simulink model "sdrzQPSKRxFPGA"  (R2016a)
settings: Solver=FixedStepDiscrete  SolverMode=SingleTasking  StartTime=0.0  StopTime=Inf  RelTol=1e-3
PreLoadFcn:
  | sdrzQPSKrxFPGA = sdrzQPSKRxFPGA_init;
InitFcn:
  | sdrzQPSKrxFPGA = sdrzQPSKRxFPGA_init;
libraries: hdlsllib x4, dspsigops x2, simulink x2, sdrzblksprivate x1, commsequence2 x1, dspmathops x1, commdigbbndpm3 x1, dspmlti4 x1, sdrzlib x1
CloseFcn:
  | clear sdrzQPSKrxFPGA;
Description:
  | This model is used to generate a targeted .bit for an SDR platform
settings Model: FPTRunName=Active  ModifiedByFormat=The MathWorks Inc.  SimulationMode=accelerator  Creator=The MathWorks, Inc.  LastModifiedBy=The MathWorks Inc.
settings DataIOCC: LimitDataPoints=on  SaveFormat=Structure  SaveOutput=off  SignalLogging=off  DSMLogging=off  SaveTime=off
settings OptimizationCC: BlockReduction=off  ConditionallyExecuteInputs=off  DefaultParameterBehavior=Inlined  ExpressionDepthLimit=2147483647  LocalBlockOutputs=off  SimCompilerOptimization=on
settings DebuggingCC: AlgebraicLoopMsg=error  UnderspecifiedInitializationDetection=Classic  MergeDetectMultiDrivingBlocksExec=none  SolverPrmCheckMsg=warning  MultiTaskDSMMsg=warning  MultiTaskCondExecSysMsg=none  SingleTaskRateTransMsg=error  ParameterPrecisionLossMsg=none  FcnCallInpInsideContextMsg=UseLocalSettings  AllowSymbolicDim=off  StateNameClashWarn=warning
settings HardwareCC: ProdBitPerPointer=32  ProdLargestAtomicFloat=None  ProdIntDivRoundTo=Undefined  ProdEndianess=Unspecified  ProdWordSize=32  ProdHWDeviceType=ASIC/FPGA->ASIC/FPGA  TargetBitPerPointer=64  TargetLongLongMode=on  TargetIntDivRoundTo=Zero  TargetEndianess=LittleEndian  TargetWordSize=64  TargetHWDeviceType=MATLAB Host  ProdEqTarget=off
settings ModelReferenceCC: PropagateSignalLabelsOutOfModel=off
settings RTWCC: CustomSourceCode=|
  | #include <stdio.h>
  | #include <stdlib.h>
settings GRTTargetCC: CombineOutputUpdateFcns=off  GRTInterface=on
settings ConfigComp: CovModelRefEnable=Off  CovSFcnEnable=off

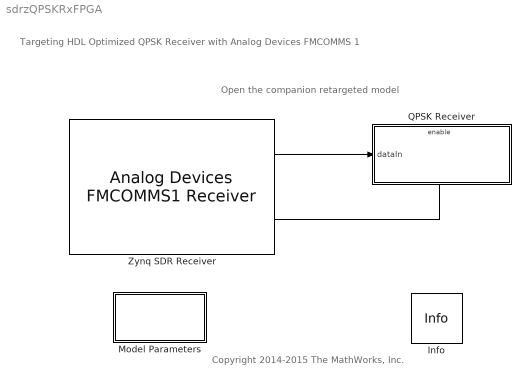
== system sdrzQPSKRxFPGA ==
  note: Copyright 2014-2015 The MathWorks, Inc.
  note: Targeting HDL Optimized QPSK Receiver with Analog Devices FMCOMMS 1
  note: Open the companion retargeted model
  Info : sdrzblksprivate/Info  SystemSampleTime=-1
  Model Parameters : Subsystem  mask(Model Parameters){SettingCtrl=Automatic gain control settings, AutoGainCtrlLoopGain=0.1, AutoGainCtrlMaxGain=400, FineFreqNormalizedLoopBW=0.06, FineFreqDampingFactor=2.5, TimeRecNormalizedLoopBW=0.01, TimeRecDampingFactor=1, DataDecThreshold=16}
      mask prompts: SettingCtrl "Setting type:"; AutoGainCtrlLoopGain "Loop gain:"; AutoGainCtrlMaxGain "Gain upper limit:"; FineFreqNormalizedLoopBW "Normalized loop bandwidth:"; FineFreqDampingFactor "Damping factor:"; TimeRecNormalizedLoopBW "Normalized loop bandwidth:"; TimeRecDampingFactor "Damping factor:"; DataDecThreshold "Threshold for the modulus of the Matched Filter ouput:"
      mask help: Set parameters for the QPSK receiver model
      mask init:
      | myException = sdrzQPSKRxFPGA_mask(gcb, 'init');
      | if ~isempty(myException)
      |    errordlg(myException.msg);
      | end
      mask TypeOptions SettingCtrl: Automatic gain control settings | Fine frequency compensation settings | Timing recovery settings | Data decoding settings
      mask Callback SettingCtrl: sdrzQPSKRxFPGA_mask(gcbh, 'cbShowHideSettingOptions');
      mask Display: disp('Model\nParameters');
  QPSK Receiver : Subsystem
      mask Display: disp('QPSK Receiver')
  Zynq SDR Receiver : sdrzlib/Analog Devices FMCOMMS1 Receiver  SourceLibraryInfo="This block requires Communications System Toolbox Support Package for Xilinx FPGA-Based Radio. <a href=\"http://www.mathworks.com/hardware-support-packages\">More information</a>"  sobjType=comm.SDRZynqFMCOMMS1Receiver  IPAddress=192.168.3.2  dataUDPPort=-1  ctrlUDPPort=-1  subDeviceList=comm.SDRZynqFMCOMMS1Receiver  sdrBlockType=SDRBlockTypeSLT.SDRRxBlock  requester=UNUSED_BY_SFCN  sdrExecutionMode=HW  LostSamplesOutputPort=off  OutputDataType=double  FrameLength=sdrzQPSKrxFPGA.Upsampling*sdrzQPSKrxFPGA.FrameSize*sdrzQPSKrxFPGA.RxBufferedFrames  EnableBurstMode=on  NumFramesInBurst=500  BypassUserLogic=on  DecimatorSelect=DDC decimator  SourceSelect=RF data  SineAmplitude=16000  SineFrequency=30000  EnableInternalClock=off  BypassIQBalance=on  CenterFrequencySource=Dialog  CenterFrequency=sdrzQPSKrxFPGA.RadioCenterFrequency  IntermediateFrequencySource=Dialog  IntermediateFrequency=sdrzQPSKrxFPGA.RadioIntermediateFrequency  IFBandwidthSource=Dialog  IFBandwidth=40e6  ADCRateSource=Dialog  ADCRate=sdrzQPSKrxFPGA.RadioADCRate  GainSource=Dialog  Gain=sdrzQPSKrxFPGA.RadioGain  DecimationFactorSource=Dialog  DecimationFactor=sdrzQPSKrxFPGA.RadioDecimationFactor  RFFrequencyIsTunable=logical(0)  SampleTime=sdrzQPSKrxFPGA.Ts  BypassDCBlockingFilter=off  IQBalanceCoefficients=64  SkipAllHardwareResetAndInitialization=off  EnableIQCalibrationTable=on  CacheIQCalibrationTable=off
  wires:
  Zynq SDR Receiver/1 -> QPSK Receiver/1(dataIn)
  Zynq SDR Receiver/2 -> QPSK Receiver/Enable

== system sdrzQPSKRxFPGA/Model Parameters ==

== system sdrzQPSKRxFPGA/QPSK Receiver ==
  dataIn : Inport  OutDataTypeStr=double
  Enable : EnablePort
  " " : MATLAB Function  TreatAsAtomicUnit=on
  Buffer1 : Buffer  N=4000  TreatMby1Signals=One channel  OutputFrames=off
  Data Type Conversion1 : DataTypeConversion  OutDataTypeStr=fixdt(1,16,15)
  Descramble and Print : Subsystem  TreatAsAtomicUnit=on
  HDLRx : Subsystem
  Unbuffer : Unbuffer  SampleBasedProcessing=Same as frame based
  Unpack FPGA Outputs : Subsystem
  wires:
  dataIn/1 -> Data Type Conversion1/1
  Unpack FPGA Outputs/2(bit2) -> " "/2(bit2)
  Unpack FPGA Outputs/1(bit1) -> " "/1(bit1)
  Unpack FPGA Outputs/3(dValid) -> " "/3(datavld)
  Buffer1/1 -> Unpack FPGA Outputs/1(In1)
  HDLRx/1(out) -> Buffer1/1
  Data Type Conversion1/1 -> Unbuffer/1
  Unbuffer/1 -> HDLRx/1(dataIn)
  " "/1(RxGo) -> Descramble and Print/Enable
  " "/2(framed_data) -> Descramble and Print/1(In1)

== system sdrzQPSKRxFPGA/QPSK Receiver/Descramble and Print ==
  In1 : Inport
  Enable : EnablePort
  BitsToDecimal1 : MATLAB Function  TreatAsAtomicUnit=on
  Buffer : Buffer  N=200  TreatMby1Signals=One channel  OutputFrames=off
  Descrambling : Subsystem
      mask Display: disp('Descrambling')
  wires:
  Descrambling/1(Out) -> BitsToDecimal1/1(u)
  In1/1 -> Buffer/1
  Buffer/1 -> Descrambling/1(In)

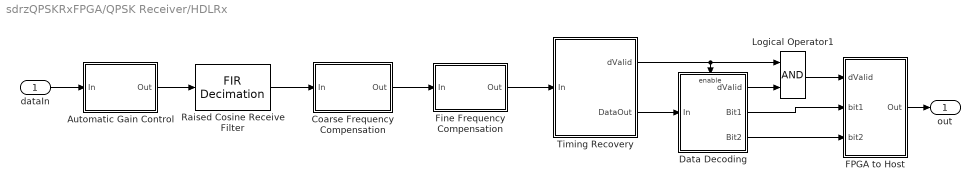
== system sdrzQPSKRxFPGA/QPSK Receiver/HDLRx ==
  dataIn : Inport
  Automatic Gain Control : Subsystem  mask{AGCLoopGain=0.1, AGCUpperLimit=400, AGCRef=1/sqrt(sdrzQPSKrxFPGA.Upsampling)}
      mask prompts: AGCLoopGain "Loop Gain"; AGCUpperLimit "Maximum Gain"; AGCRef "Desired Amplitude"
  Coarse Frequency Compensation : Subsystem
  Data Decoding : Subsystem  TreatAsAtomicUnit=on  mask{Threshold=16}
      mask help:
      | Package synchronization is achieved by correlating (matched filtering) the Barker codes with the streams given by the Timing Recovery subsystem.
      | We deem successful package synchronization if the modulus of the matched filter output exceeds the threshold value defined below.
  FPGA to Host : Subsystem
  Fine Frequency Compensation : Subsystem
  Logical Operator1 : Logic  AllPortsSameDT=off  OutDataTypeStr=boolean
  Raised Cosine Receive Filter : dspmlti4/FIR Decimation  FilterSource=Dialog parameters  h=sdrzQPSKrxFPGA.ReceiverFilterCoefficients  D=sdrzQPSKrxFPGA.Upsampling/sdrzQPSKrxFPGA.Downsampling  filtStruct=Direct form  FilterObject=Hm_firdecim  framing=Allow multirate processing  inputOffset=0  outputBufInitCond=0  roundingMode=Floor  overflowMode=off  firstCoeffDataTypeStr=Inherit: Same word length as input  firstCoeffMin=[]  firstCoeffMax=[]  firstCoeffLastDataTypeStr=Inherit: Same word length as input  outputMode=Binary point scaling  outputWordLength=16  outputFracLength=14  outputDataTypeStr=fixdt(1,16,14)  outputMin=[]  outputMax=[]  outputLastDataTypeStr=fixdt(1,16,14)
  Timing Recovery : Subsystem
  out : Outport
  wires:
  Timing Recovery/2(DataOut) -> Data Decoding/1(In)
  dataIn/1 -> Automatic Gain Control/1(In)
  Fine Frequency Compensation/1(Out) -> Timing Recovery/1(In)
  Coarse Frequency Compensation/1(Out) -> Fine Frequency Compensation/1(In)
  Timing Recovery/1(dValid) -> Logical Operator1/1, Data Decoding/Enable
  Data Decoding/1(dValid) -> Logical Operator1/2
  Raised Cosine Receive Filter/1 -> Coarse Frequency Compensation/1(In)
  Automatic Gain Control/1(Out) -> Raised Cosine Receive Filter/1
  Logical Operator1/1 -> FPGA to Host/1(dValid)
  Data Decoding/3(Bit2) -> FPGA to Host/3(bit2)
  Data Decoding/2(Bit1) -> FPGA to Host/2(bit1)
  FPGA to Host/1(Out) -> out/1

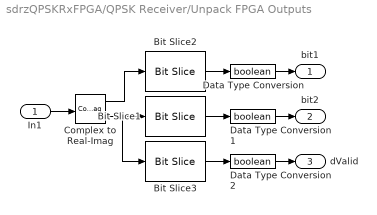
== system sdrzQPSKRxFPGA/QPSK Receiver/Unpack FPGA Outputs ==
  In1 : Inport
  Bit Slice1 : hdlsllib/HDL Operations/Bit Slice  lidx=0  ridx=0
  Bit Slice2 : hdlsllib/HDL Operations/Bit Slice  lidx=0  ridx=0
  Bit Slice3 : hdlsllib/HDL Operations/Bit Slice  lidx=15  ridx=15
  Complex to Real-Imag : ComplexToRealImag
  Data Type Conversion : DataTypeConversion  OutDataTypeStr=boolean
  Data Type Conversion1 : DataTypeConversion  OutDataTypeStr=boolean
  Data Type Conversion2 : DataTypeConversion  OutDataTypeStr=boolean
  bit1 : Outport
  bit2 : Outport  Port=2
  dValid : Outport  Port=3
  wires:
  In1/1 -> Complex to Real-Imag/1
  Complex to Real-Imag/1 -> Bit Slice2/1
  Complex to Real-Imag/2 -> Bit Slice3/1, Bit Slice1/1
  Bit Slice2/1 -> Data Type Conversion/1
  Bit Slice1/1 -> Data Type Conversion1/1
  Bit Slice3/1 -> Data Type Conversion2/1
  Data Type Conversion/1 -> bit1/1
  Data Type Conversion1/1 -> bit2/1
  Data Type Conversion2/1 -> dValid/1

== system sdrzQPSKRxFPGA/QPSK Receiver/Descramble and Print/Descrambling ==
  In : Inport
  Descrambler : commsequence2/Descrambler  M=2  poly=[1 1 1 0 1]  iniStaSource=Dialog Parameter  ini_sta=[0 0 0 0]  resetViaPort=off
  Selector : Selector  IndexOptions=Index vector (dialog)  Indices=[sdrzQPSKrxFPGA.BarkerLength*log2(sdrzQPSKrxFPGA.M)+1:sdrzQPSKrxFPGA.FrameSize*log2(sdrzQPSKrxFPGA.M)]  OutputSizes=1
  Selector1 : Selector  IndexOptions=Index vector (dialog)  Indices=[1:sdrzQPSKrxFPGA.MsgLength]  OutputSizes=1
  Out : Outport
  wires:
  Descrambler/1 -> Selector1/1
  Selector1/1 -> Out/1
  In/1 -> Selector/1
  Selector/1 -> Descrambler/1

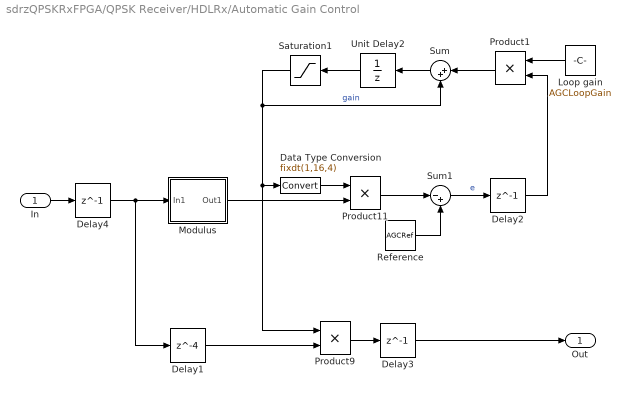
== system sdrzQPSKRxFPGA/QPSK Receiver/HDLRx/Automatic Gain Control ==
  In : Inport
  Data Type Conversion : DataTypeConversion  OutDataTypeStr=fixdt(1,16,4)  SaturateOnIntegerOverflow=on
  Delay1 : Delay  DelayLength=4  InitialCondition=0
  Delay2 : Delay  DelayLength=1  InitialCondition=0
  Delay3 : Delay  DelayLength=1  InitialCondition=0
  Delay4 : Delay  DelayLength=1  InitialCondition=0
  Loop gain : Constant  Value=AGCLoopGain  OutDataTypeStr=fixdt(1,16,10)  SampleTime=sdrzQPSKrxFPGA.Ts
  Modulus : Subsystem
  Product1 : Product  OutDataTypeStr=fixdt(1,16,10)  RndMeth=Zero
  Product11 : Product  OutDataTypeStr=fixdt(1,16,10)  RndMeth=Zero
  Product9 : Product  OutDataTypeStr=fixdt(1,16,14)  SaturateOnIntegerOverflow=on  RndMeth=Zero
  Reference : Constant  Value=AGCRef  OutDataTypeStr=fixdt(1,16,10)  SampleTime=sdrzQPSKrxFPGA.Ts
  Saturation1 : Saturate  UpperLimit=AGCUpperLimit  LowerLimit=1e-5
  Sum : Sum  Inputs=|++  OutDataTypeStr=fixdt(1,23,10)  SaturateOnIntegerOverflow=on
  Sum1 : Sum  Inputs=|-+  OutDataTypeStr=Inherit: Same as first input
  Unit Delay2 : UnitDelay  SampleTime=-1
  Out : Outport  PortDimensions=1
  wires:
  In/1 -> Delay4/1
  Product11/1 -> Sum1/1
  Data Type Conversion/1 -> Product11/1
  Reference/1 -> Sum1/2
  Sum/1 -> Unit Delay2/1
  Sum1/1 -> Delay2/1  "e"
  Product9/1 -> Delay3/1
  Delay1/1 -> Product9/2
  Delay3/1 -> Out/1
  Delay2/1 -> Product1/2
  Unit Delay2/1 -> Saturation1/1
  Delay4/1 -> Delay1/1, Modulus/1(In1)
  Modulus/1(Out1) -> Product11/2
  Product1/1 -> Sum/1
  Loop gain/1 -> Product1/1
  Saturation1/1 -> Sum/2, Data Type Conversion/1, Product9/1  "gain"

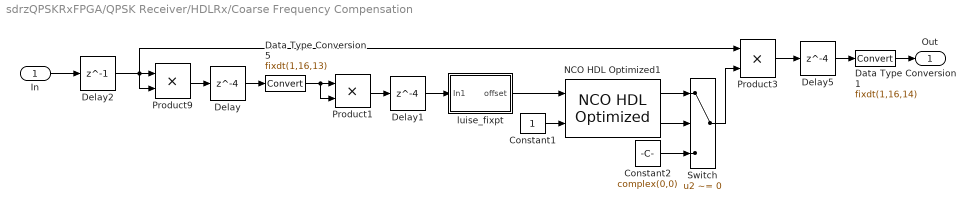
== system sdrzQPSKRxFPGA/QPSK Receiver/HDLRx/Coarse Frequency Compensation ==
  In : Inport  PortDimensions=1
  Constant1 : Constant  OutDataTypeStr=boolean  SampleTime=sdrzQPSKrxFPGA.Ts*sdrzQPSKrxFPGA.Upsampling/sdrzQPSKrxFPGA.Downsampling
  Constant2 : Constant  Value=complex(0,0)  OutDataTypeStr=fixdt(1,10,8)  SampleTime=sdrzQPSKrxFPGA.Ts*sdrzQPSKrxFPGA.Upsampling/sdrzQPSKrxFPGA.Downsampling
  Data Type Conversion1 : DataTypeConversion  OutDataTypeStr=fixdt(1,16,14)
  Data Type Conversion5 : DataTypeConversion  OutDataTypeStr=fixdt(1,16,13)  SaturateOnIntegerOverflow=on
  Delay : Delay  DelayLength=4  InitialCondition=0
  Delay1 : Delay  DelayLength=4  InitialCondition=0
  Delay2 : Delay  DelayLength=1  InitialCondition=0
  Delay5 : Delay  DelayLength=4  InitialCondition=0
  NCO HDL Optimized1 : dspsigops/NCO HDL Optimized  PhaseIncrementSource=Input port  PhaseIncrement=100  PhaseOffsetSource=Property  PhaseOffset=0  DitherSource=None  NumDitherBits=1  PhaseQuantization=on  NumQuantizerAccumulatorBits=16  LUTCompress=on  ResetAction=off  ValidInputPort=on  Waveform=Complex exponential  PhasePort=off  AccumulatorWL=17  OutputDataType=Binary point scaling  OutputWL=10  OutputFL=8  SimulateUsing=Code generation
  Product1 : Product  SaturateOnIntegerOverflow=on  RndMeth=Zero
  Product3 : Product  SaturateOnIntegerOverflow=on  RndMeth=Zero
  Product9 : Product  SaturateOnIntegerOverflow=on  RndMeth=Zero
  Switch : Switch  Criteria=u2 ~= 0
  luise_fixpt : Subsystem
  Out : Outport
  wires:
  Data Type Conversion1/1 -> Out/1
  Delay1/1 -> luise_fixpt/1(In1)
  Product9/1 -> Delay/1
  Delay/1 -> Data Type Conversion5/1
  Data Type Conversion5/1 -> Product1/1, Product1/2
  Product1/1 -> Delay1/1
  In/1 -> Delay2/1
  Product3/1 -> Delay5/1
  Delay5/1 -> Data Type Conversion1/1
  Constant1/1 -> NCO HDL Optimized1/2
  NCO HDL Optimized1/2 -> Switch/2
  NCO HDL Optimized1/1 -> Switch/1
  Constant2/1 -> Switch/3
  Switch/1 -> Product3/2
  Delay2/1 -> Product3/1, Product9/2, Product9/1
  luise_fixpt/1(offset) -> NCO HDL Optimized1/1

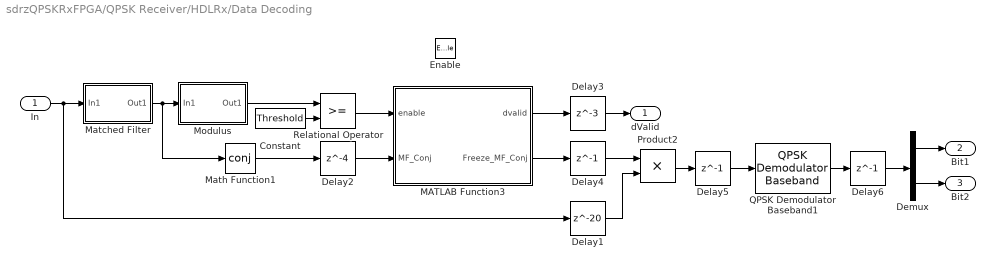
== system sdrzQPSKRxFPGA/QPSK Receiver/HDLRx/Data Decoding ==
  In : Inport
  Enable : EnablePort
  Constant : Constant  Value=Threshold  OutDataTypeStr=Inherit: Inherit via back propagation  SampleTime=sdrzQPSKrxFPGA.Ts*sdrzQPSKrxFPGA.Upsampling/sdrzQPSKrxFPGA.Downsampling
  Delay1 : Delay  DelayLength=20  InitialCondition=0
  Delay2 : Delay  DelayLength=4  InitialCondition=0
  Delay3 : Delay  DelayLength=3  InitialCondition=0
  Delay4 : Delay  DelayLength=1  InitialCondition=0
  Delay5 : Delay  DelayLength=1  InitialCondition=0
  Delay6 : Delay  DelayLength=1  InitialCondition=0
  Demux : Demux  Outputs=2
  MATLAB Function3 : MATLAB Function  TreatAsAtomicUnit=on
  Matched Filter : Subsystem
  Math Function1 : Math  Operator=conj  OutputSignalType=complex  SaturateOnIntegerOverflow=on
  Modulus : Subsystem
  Product2 : Product  SaturateOnIntegerOverflow=on  RndMeth=Zero
  QPSK Demodulator Baseband1 : commdigbbndpm3/QPSK Demodulator Baseband  OutType=Bit  DecType=Hard decision  VarSource=Dialog  Variance=1  Dec=Gray  Ph=pi/4  outDtype1=boolean  outDtype2=Inherit via internal rule  derotateFactorWordLen=16  derotateFactorDataTypeStr=Inherit: Same word length as input  derotateFactorLastDataTypeStr=Inherit: Same word length as input
  Relational Operator : RelationalOperator  OutDataTypeStr=boolean  InputSameDT=on
  dValid : Outport  InitialOutput=0
  Bit1 : Outport  Port=2  InitialOutput=0
  Bit2 : Outport  Port=3  InitialOutput=0
  wires:
  Demux/2 -> Bit2/1
  Demux/1 -> Bit1/1
  Delay3/1 -> dValid/1
  Delay6/1 -> Demux/1
  Delay5/1 -> QPSK Demodulator Baseband1/1
  Delay1/1 -> Product2/2
  Delay4/1 -> Product2/1
  Delay2/1 -> MATLAB Function3/2(MF_Conj)
  Matched Filter/1(Out1) -> Math Function1/1, Modulus/1(In1)
  In/1 -> Delay1/1, Matched Filter/1(In1)
  Product2/1 -> Delay5/1
  Relational Operator/1 -> MATLAB Function3/1(enable)
  Math Function1/1 -> Delay2/1
  MATLAB Function3/2(Freeze_MF_Conj) -> Delay4/1
  MATLAB Function3/1(dvalid) -> Delay3/1
  QPSK Demodulator Baseband1/1 -> Delay6/1
  Modulus/1(Out1) -> Relational Operator/1
  Constant/1 -> Relational Operator/2

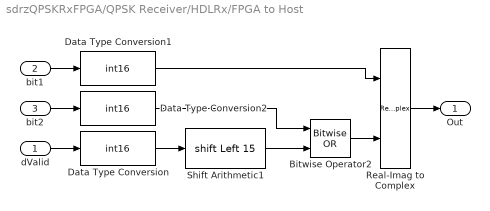
== system sdrzQPSKRxFPGA/QPSK Receiver/HDLRx/FPGA to Host ==
  dValid : Inport
  bit1 : Inport  Port=2
  bit2 : Inport  Port=3
  Bitwise Operator2 : simulink/Logic and Bit Operations/Bitwise Operator  logicop=OR  UseBitMask=off  NumInputPorts=2  BitMask=bin2dec('11011001')  BitMaskRealWorld=Stored Integer
  Data Type Conversion : DataTypeConversion  OutDataTypeStr=int16
  Data Type Conversion1 : DataTypeConversion  OutDataTypeStr=int16
  Data Type Conversion2 : DataTypeConversion  OutDataTypeStr=int16
  Real-Imag to Complex : RealImagToComplex
  Shift Arithmetic1 : ArithShift  BitShiftNumber=15  BitShiftDirection=Left
  Out : Outport
  wires:
  Data Type Conversion2/1 -> Bitwise Operator2/1
  Data Type Conversion1/1 -> Real-Imag to Complex/1
  Data Type Conversion/1 -> Shift Arithmetic1/1
  Real-Imag to Complex/1 -> Out/1
  bit2/1 -> Data Type Conversion2/1
  dValid/1 -> Data Type Conversion/1
  Bitwise Operator2/1 -> Real-Imag to Complex/2
  Shift Arithmetic1/1 -> Bitwise Operator2/2
  bit1/1 -> Data Type Conversion1/1

== system sdrzQPSKRxFPGA/QPSK Receiver/HDLRx/Fine Frequency Compensation ==
  In : Inport  PortDimensions=1
  Delay2 : Delay  DelayLength=1  InitialCondition=0
  Delay5 : Delay  DelayLength=9  InitialCondition=0
  Loop Filter : Subsystem  mask{BnTs=0.06, zeta=2.5, N=sdrzQPSKrxFPGA.Upsampling/sdrzQPSKrxFPGA.Downsampling, Kp=sdrzQPSKrxFPGA.FineFreqPEDGain, K0=sdrzQPSKrxFPGA.FineFreqCompensateGain}
      mask prompts: BnTs "Normalized Loop Bandwidth"; zeta "Damping Factor"; N "Number of Samples/Symbol"; Kp "Phase Detector Gain (Kp)"; K0 "DDS Gain (K0)"
      mask init:
      | % See C.57 to C.61 in Michael Rice's "Digital Communications 
      | % - A Discrete-Time Approach" for details
      | theta = BnTs/(zeta+0.25/zeta)/N;
      | d = 1 + 2*zeta*theta + theta*theta;
      | K1 = 4*zeta*theta/d;
      | K2 = 4*theta*theta/d;
      | K1 = K1/(Kp*K0);
      | K2 = K2/(Kp*K0);
      mask Display: disp('Loop Filter')
  MATLAB Function1 : MATLAB Function  TreatAsAtomicUnit=on
  NCO : Subsystem
  Product9 : Product  OutDataTypeStr=fixdt(1,16,14)  SaturateOnIntegerOverflow=on  RndMeth=Zero
  Out : Outport
  wires:
  In/1 -> Delay5/1
  Delay5/1 -> Product9/1
  Product9/1 -> Delay2/1
  MATLAB Function1/1(e) -> Loop Filter/1(e)
  NCO/1(Out1) -> Product9/2
  Delay2/1 -> Out/1, MATLAB Function1/1(In)
  Loop Filter/1(v) -> NCO/1(In1)

== system sdrzQPSKRxFPGA/QPSK Receiver/HDLRx/Timing Recovery ==
  In : Inport
  Delay5 : Delay  DelayLength=6
  Integer Delay3 : Delay  DelayLength=1  InputProcessing=Inherited
  Integer Delay4 : Delay  DelayLength=1  InputProcessing=Inherited
  Interpolation Control : MATLAB Function
  Interpolation Filter : Subsystem
  Loop Filter : Subsystem  mask{BnTs=0.01, zeta=1, Kp=sdrzQPSKrxFPGA.TimingRecTEDGain, K0=sdrzQPSKrxFPGA.TimingRecCompensateGain, N=sdrzQPSKrxFPGA.Upsampling/sdrzQPSKrxFPGA.Downsampling}
      mask prompts: BnTs "Loop Bandwidth"; zeta "Loop Damping Factor"; Kp "Phase Detector Gain (Kp)"; K0 "DDS gain (K0)"; N "Number of Samples/symbol (N)"
      mask init:
      | % See C.57 to C.61 in Michael Rice's "Digital Communications 
      | % - A Discrete-Time Approach" for details
      | theta = BnTs/(zeta+0.25/zeta)/N;
      | d = 1 + 2*zeta*theta + theta*theta;
      | K1 = 4*zeta*theta/d;
      | K2 = 4*theta*theta/d;
      | K1 = K1/(Kp*K0);
      | K2 = K2/(Kp*K0);
      mask Display: disp('Loop Filter');
  Timing Error Detector : MATLAB Function  TreatAsAtomicUnit=on
  dValid : Outport
  DataOut : Outport  Port=2
  wires:
  Interpolation Filter/1(Out) -> Timing Error Detector/1(In), DataOut/1
  In/1 -> Delay5/1
  Integer Delay4/1 -> Interpolation Filter/2(mu)
  Interpolation Control/2(mu) -> Integer Delay4/1
  Interpolation Control/1(Underflow) -> Integer Delay3/1
  Delay5/1 -> Interpolation Filter/1(In)
  Integer Delay3/1 -> Timing Error Detector/2(strobe), dValid/1
  Timing Error Detector/1(e) -> Loop Filter/1(e)
  Loop Filter/1(v) -> Interpolation Control/1(Delta)

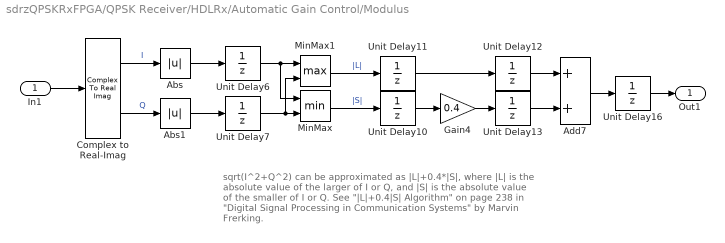
== system sdrzQPSKRxFPGA/QPSK Receiver/HDLRx/Automatic Gain Control/Modulus ==
  note: sqrt(I^2+Q^2) can be approximated as |L|+0.4*|S|,
      | where |L| is the absolute value of the larger of I or Q,
      | and |S| is the absolute value of the smaller of I or Q.
      |
      | See "|L|+0.4|S| Algorithm" on page 238 in "Digital Signal
      | Processing in Communication Systems" by Marvin Frerking.
  In1 : Inport
  Abs : Abs
  Abs1 : Abs
  Add7 : Sum
  Complex to Real-Imag : ComplexToRealImag
  Gain4 : Gain  Gain=0.4  OutDataTypeStr=fixdt(1,16,15)
  MinMax : MinMax  Inputs=2
  MinMax1 : MinMax  Function=max  Inputs=2
  Unit Delay{6..7,10..13,16} (7 alike) : UnitDelay  SampleTime=-1
  Out1 : Outport
  wires:
  Unit Delay11/1 -> Unit Delay12/1
  Unit Delay16/1 -> Out1/1
  Unit Delay10/1 -> Gain4/1
  Unit Delay12/1 -> Add7/1
  Abs1/1 -> Unit Delay7/1
  Add7/1 -> Unit Delay16/1
  Abs/1 -> Unit Delay6/1
  Complex to Real-Imag/1 -> Abs/1  "I"
  Complex to Real-Imag/2 -> Abs1/1  "Q"
  MinMax1/1 -> Unit Delay11/1  "|L|"
  Unit Delay13/1 -> Add7/2
  Gain4/1 -> Unit Delay13/1
  MinMax/1 -> Unit Delay10/1  "|S|"
  Unit Delay6/1 -> MinMax/1, MinMax1/1
  Unit Delay7/1 -> MinMax1/2, MinMax/2
  In1/1 -> Complex to Real-Imag/1

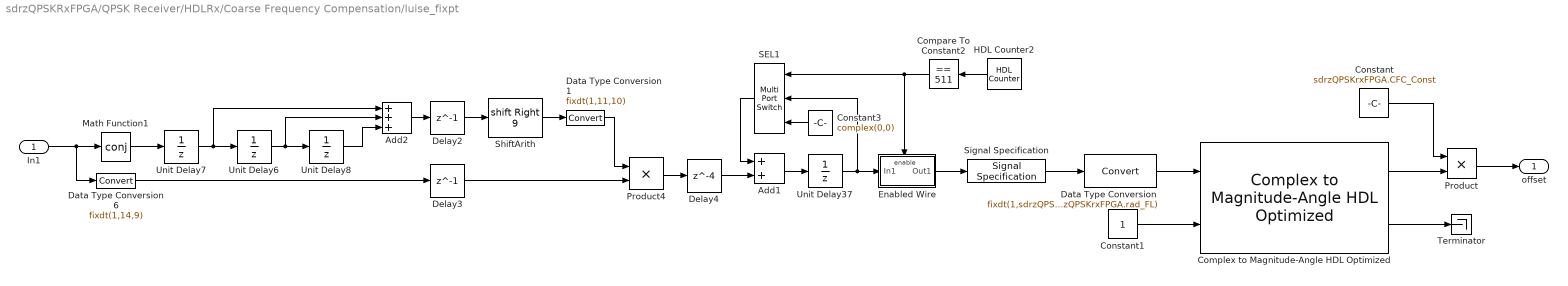
== system sdrzQPSKRxFPGA/QPSK Receiver/HDLRx/Coarse Frequency Compensation/luise_fixpt ==
  In1 : Inport
  Add1 : Sum  OutDataTypeStr=fixdt(1,33,20)
  Add2 : Sum  Inputs=+++  OutDataTypeStr=fixdt(1,33,20)
  Compare To Constant2 : simulink/Logic and Bit Operations/Compare To Constant  relop===  const=511  OutDataTypeStr=boolean
  Complex to Magnitude-Angle HDL Optimized : dspmathops/Complex to Magnitude-Angle HDL Optimized  NumIterationsSource=Property  NumIterations=5  OutputFormat=Angle  AngleFormat=Normalized  ScaleOutput=on  SimulateUsing=Code generation
  Constant : Constant  Value=sdrzQPSKrxFPGA.CFC_Const  OutDataTypeStr=int16  SampleTime=sdrzQPSKrxFPGA.Ts*sdrzQPSKrxFPGA.Upsampling/sdrzQPSKrxFPGA.Downsampling
  Constant1 : Constant  OutDataTypeStr=boolean  SampleTime=sdrzQPSKrxFPGA.Ts*sdrzQPSKrxFPGA.Upsampling/sdrzQPSKrxFPGA.Downsampling
  Constant3 : Constant  Value=complex(0,0)  OutDataTypeStr=fixdt(1,16,14)  SampleTime=sdrzQPSKrxFPGA.Ts*sdrzQPSKrxFPGA.Upsampling/sdrzQPSKrxFPGA.Downsampling
  Data Type Conversion : DataTypeConversion  OutDataTypeStr=fixdt(1,sdrzQPSKrxFPGA.rad_WL,sdrzQPSKrxFPGA.rad_FL)
  Data Type Conversion1 : DataTypeConversion  OutDataTypeStr=fixdt(1,11,10)
  Data Type Conversion6 : DataTypeConversion  OutDataTypeStr=fixdt(1,14,9)  SaturateOnIntegerOverflow=on
  Delay2 : Delay  DelayLength=1  InitialCondition=0
  Delay3 : Delay  DelayLength=1  InitialCondition=0
  Delay4 : Delay  DelayLength=4  InitialCondition=0
  Enabled Wire : Subsystem  TreatAsAtomicUnit=on
  HDL Counter2 : hdlsllib/HDL Operations/HDL Counter  CountType=Count limited  CountInit=0  CountStep=1  CountMax=511  CountFromType=Initial value  CountFrom=0  CountResetPort=off  CountLoadPort=off  CountEnbPort=off  CountDirPort=off  CountDataType=Unsigned  CountWordLen=9  CountFracLen=0  CountSampTime=-1
  Math Function1 : Math  Operator=conj  OutputSignalType=complex  SaturateOnIntegerOverflow=on
  Product : Product  OutDataTypeStr=int16
  Product4 : Product  SaturateOnIntegerOverflow=on  RndMeth=Zero
  SEL1 : MultiPortSwitch  DataPortOrder=Zero-based contiguous  Inputs=2  DiagnosticForDefault=None  OutDataTypeStr=fixdt(1,33,20)
  ShiftArith : ArithShift  BitShiftNumber=9  BitShiftDirection=Right
  Signal Specification : SignalSpecification  Dimensions=1
  Terminator : Terminator
  Unit Delay37 : UnitDelay  InitialCondition=0+0j  SampleTime=-1
  Unit Delay6 : UnitDelay  SampleTime=-1
  Unit Delay7 : UnitDelay  SampleTime=-1
  Unit Delay8 : UnitDelay  SampleTime=-1
  offset : Outport  PortDimensions=1
  wires:
  Delay2/1 -> ShiftArith/1
  Delay3/1 -> Product4/2
  ShiftArith/1 -> Data Type Conversion1/1
  Unit Delay8/1 -> Add2/3
  HDL Counter2/1 -> Compare To Constant2/1
  Compare To Constant2/1 -> Enabled Wire/Enable, SEL1/1
  Unit Delay7/1 -> Unit Delay6/1, Add2/1
  Unit Delay6/1 -> Add2/2, Unit Delay8/1
  Constant3/1 -> SEL1/3
  Data Type Conversion6/1 -> Delay3/1
  Add2/1 -> Delay2/1
  SEL1/1 -> Add1/1
  Unit Delay37/1 -> Enabled Wire/1(In1), SEL1/2
  Delay4/1 -> Add1/2
  Data Type Conversion1/1 -> Product4/1
  In1/1 -> Data Type Conversion6/1, Math Function1/1
  Product4/1 -> Delay4/1
  Math Function1/1 -> Unit Delay7/1
  Add1/1 -> Unit Delay37/1
  Enabled Wire/1(Out1) -> Signal Specification/1
  Product/1 -> offset/1
  Constant/1 -> Product/1
  Complex to Magnitude-Angle HDL Optimized/1 -> Product/2
  Constant1/1 -> Complex to Magnitude-Angle HDL Optimized/2
  Signal Specification/1 -> Data Type Conversion/1
  Complex to Magnitude-Angle HDL Optimized/2 -> Terminator/1
  Data Type Conversion/1 -> Complex to Magnitude-Angle HDL Optimized/1

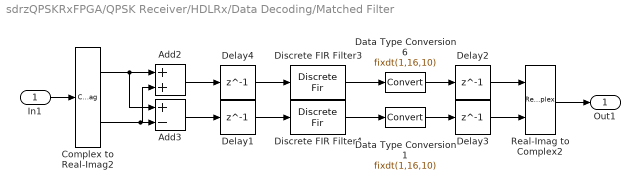
== system sdrzQPSKRxFPGA/QPSK Receiver/HDLRx/Data Decoding/Matched Filter ==
  In1 : Inport
  Add2 : Sum
  Add3 : Sum  Inputs=+-
  Complex to Real-Imag2 : ComplexToRealImag
  Data Type Conversion1 : DataTypeConversion  OutDataTypeStr=fixdt(1,16,10)
  Data Type Conversion6 : DataTypeConversion  OutDataTypeStr=fixdt(1,16,10)
  Delay{1..4} (4 alike) : Delay  DelayLength=1  InitialCondition=0
  Discrete FIR Filter3 : DiscreteFir  FilterStructure=Direct form transposed  Coefficients=[-1 1 -1 1 -1 -1 1 1 -1 -1 -1 -1 -1]
  Discrete FIR Filter4 : DiscreteFir  FilterStructure=Direct form transposed  Coefficients=-1*[-1 1 -1 1 -1 -1 1 1 -1 -1 -1 -1 -1]
  Real-Imag to Complex2 : RealImagToComplex
  Out1 : Outport
  wires:
  Delay1/1 -> Discrete FIR Filter4/1
  Delay3/1 -> Real-Imag to Complex2/2
  Delay2/1 -> Real-Imag to Complex2/1
  Discrete FIR Filter4/1 -> Data Type Conversion1/1
  Delay4/1 -> Discrete FIR Filter3/1
  Discrete FIR Filter3/1 -> Data Type Conversion6/1
  Add3/1 -> Delay1/1
  Data Type Conversion6/1 -> Delay2/1
  Add2/1 -> Delay4/1
  Data Type Conversion1/1 -> Delay3/1
  Complex to Real-Imag2/1 -> Add3/1, Add2/1
  Complex to Real-Imag2/2 -> Add2/2, Add3/2
  Real-Imag to Complex2/1 -> Out1/1
  In1/1 -> Complex to Real-Imag2/1

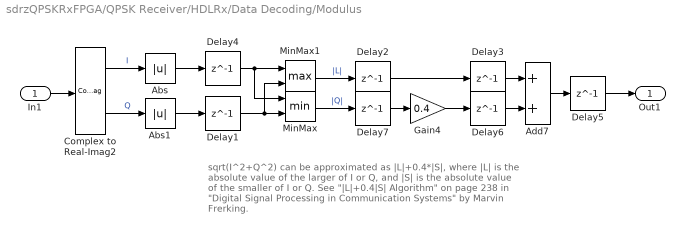
== system sdrzQPSKRxFPGA/QPSK Receiver/HDLRx/Data Decoding/Modulus ==
  note: sqrt(I^2+Q^2) can be approximated as |L|+0.4*|S|,
      | where |L| is the absolute value of the larger of I or Q,
      | and |S| is the absolute value of the smaller of I or Q.
      |
      | See "|L|+0.4|S| Algorithm" on page 238 in "Digital Signal
      | Processing in Communication Systems" by Marvin Frerking.
  In1 : Inport
  Abs : Abs
  Abs1 : Abs
  Add7 : Sum
  Complex to Real-Imag2 : ComplexToRealImag
  Delay{1..7} (7 alike) : Delay  DelayLength=1  InitialCondition=0
  Gain4 : Gain  Gain=0.4  OutDataTypeStr=fixdt(1,16,15)
  MinMax : MinMax  Inputs=2
  MinMax1 : MinMax  Function=max  Inputs=2
  Out1 : Outport
  wires:
  Complex to Real-Imag2/1 -> Abs/1  "I"
  Complex to Real-Imag2/2 -> Abs1/1  "Q"
  Delay3/1 -> Add7/1
  Delay5/1 -> Out1/1
  Delay6/1 -> Add7/2
  Delay4/1 -> MinMax/1, MinMax1/1
  Delay1/1 -> MinMax/2, MinMax1/2
  Delay2/1 -> Delay3/1
  Delay7/1 -> Gain4/1
  Add7/1 -> Delay5/1
  MinMax/1 -> Delay7/1  "|Q|"
  MinMax1/1 -> Delay2/1  "|L|"
  Gain4/1 -> Delay6/1
  Abs/1 -> Delay4/1
  Abs1/1 -> Delay1/1
  In1/1 -> Complex to Real-Imag2/1

== system sdrzQPSKRxFPGA/QPSK Receiver/HDLRx/Fine Frequency Compensation/Loop Filter ==
  note: Proportional-plus-Integrator Loop Filter,
      | Infinite DC Response to guarantee convergence
  e : Inport
  Data Type Conversion3 : DataTypeConversion  OutDataTypeStr=fixdt(1,32,29)
  Delay1 : Delay  DelayLength=1  InitialCondition=0
  Delay2 : Delay  DelayLength=1  InitialCondition=0
  Digital Filter : Subsystem
  K1 : Gain  Gain=K1
  K2 : Gain  Gain=K2
  Sum2 : Sum  OutDataTypeStr=fixdt(1,22,19)  SaturateOnIntegerOverflow=on  InputSameDT=on
  v : Outport
  wires:
  K1/1 -> Data Type Conversion3/1
  e/1 -> Delay2/1
  Delay2/1 -> K1/1, K2/1
  Data Type Conversion3/1 -> Sum2/1
  K2/1 -> Digital Filter/1(In1)
  Sum2/1 -> Delay1/1
  Digital Filter/1(Out1) -> Sum2/2
  Delay1/1 -> v/1

== system sdrzQPSKRxFPGA/QPSK Receiver/HDLRx/Fine Frequency Compensation/NCO ==
  In1 : Inport
  Constant : Constant  Value=sdrzQPSKrxFPGA.FFC_Const  OutDataTypeStr=int16  SampleTime=sdrzQPSKrxFPGA.Ts*sdrzQPSKrxFPGA.Upsampling/sdrzQPSKrxFPGA.Downsampling
  Constant1 : Constant  OutDataTypeStr=boolean  SampleTime=sdrzQPSKrxFPGA.Ts*sdrzQPSKrxFPGA.Upsampling/sdrzQPSKrxFPGA.Downsampling
  Constant2 : Constant  Value=complex(0,0)  OutDataTypeStr=fixdt(1,10,8)  SampleTime=sdrzQPSKrxFPGA.Ts*sdrzQPSKrxFPGA.Upsampling/sdrzQPSKrxFPGA.Downsampling
  Delay3 : Delay  DelayLength=1  InitialCondition=0
  NCO HDL Optimized : dspsigops/NCO HDL Optimized  PhaseIncrementSource=Input port  PhaseIncrement=100  PhaseOffsetSource=Property  PhaseOffset=0  DitherSource=None  NumDitherBits=1  PhaseQuantization=on  NumQuantizerAccumulatorBits=16  LUTCompress=on  ResetAction=off  ValidInputPort=on  Waveform=Complex exponential  PhasePort=off  AccumulatorWL=17  OutputDataType=Binary point scaling  OutputWL=10  OutputFL=8  SimulateUsing=Code generation
  Product : Product  OutDataTypeStr=int16
  Signal Specification : SignalSpecification  Dimensions=1
  Switch : Switch  Criteria=u2 ~= 0
  Out1 : Outport
  wires:
  In1/1 -> Product/1
  Constant/1 -> Product/2
  Product/1 -> Signal Specification/1
  Switch/1 -> Delay3/1
  Signal Specification/1 -> NCO HDL Optimized/1
  NCO HDL Optimized/1 -> Switch/1
  Constant1/1 -> NCO HDL Optimized/2
  NCO HDL Optimized/2 -> Switch/2
  Constant2/1 -> Switch/3
  Delay3/1 -> Out1/1

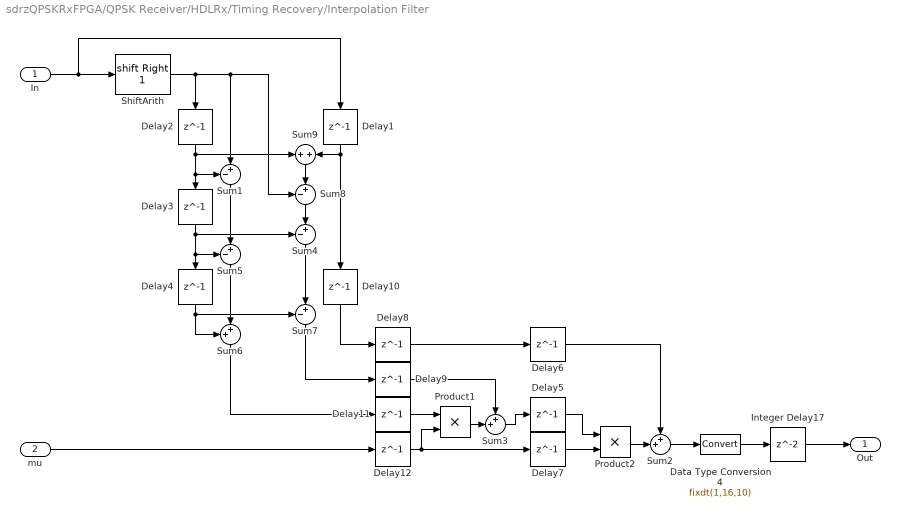
== system sdrzQPSKRxFPGA/QPSK Receiver/HDLRx/Timing Recovery/Interpolation Filter ==
  In : Inport
  mu : Inport  Port=2
  Data Type Conversion4 : DataTypeConversion  OutDataTypeStr=fixdt(1,16,10)
  Delay{1..12} (12 alike) : Delay  DelayLength=1  InitialCondition=0
  Integer Delay17 : Delay  InputProcessing=Inherited
  Product1 : Product  OutDataTypeStr=fixdt(1,16,10)  RndMeth=Zero
  Product2 : Product  RndMeth=Zero
  ShiftArith : ArithShift  BitShiftNumber=1  BitShiftDirection=Right
  Sum{1,4..5,8} (4 alike) : Sum  Inputs=-+|
  Sum2 : Sum  Inputs=++|
  Sum3 : Sum  Inputs=++|  OutDataTypeStr=fixdt(1,16,10)
  Sum6 : Sum  Inputs=++|  OutDataTypeStr=fixdt(1,16,11)  SaturateOnIntegerOverflow=on
  Sum7 : Sum  Inputs=-+|  OutDataTypeStr=fixdt(1,16,10)
  Sum9 : Sum  Inputs=+|+
  Out : Outport
  wires:
  ShiftArith/1 -> Delay2/1, Sum1/2, Sum8/1
  Delay1/1 -> Sum9/2, Delay10/1
  Delay2/1 -> Sum9/1, Delay3/1, Sum1/1
  Sum8/1 -> Sum4/2
  Delay3/1 -> Delay4/1, Sum5/1, Sum4/1
  Sum1/1 -> Sum5/2
  Delay4/1 -> Sum6/1, Sum7/1
  Sum5/1 -> Sum6/2
  Sum4/1 -> Sum7/2
  Delay5/1 -> Product2/1
  Sum3/1 -> Delay5/1
  Product2/1 -> Sum2/2
  Product1/1 -> Sum3/2
  Sum2/1 -> Data Type Conversion4/1
  Delay11/1 -> Product1/1
  Delay9/1 -> Sum3/1
  Delay8/1 -> Delay6/1
  Delay12/1 -> Delay7/1, Product1/2
  Delay7/1 -> Product2/2
  Delay6/1 -> Sum2/1
  Delay10/1 -> Delay8/1
  Sum7/1 -> Delay9/1
  Sum6/1 -> Delay11/1
  mu/1 -> Delay12/1
  Integer Delay17/1 -> Out/1
  In/1 -> Delay1/1, ShiftArith/1
  Data Type Conversion4/1 -> Integer Delay17/1
  Sum9/1 -> Sum8/2

== system sdrzQPSKRxFPGA/QPSK Receiver/HDLRx/Timing Recovery/Loop Filter ==
  note: Proportional-Plus-Integrator Loop Filter,
      | Infinite DC Response to guarantee convergence
  e : Inport
  Data Type Conversion17 : DataTypeConversion  OutDataTypeStr=fixdt(1,11,10)
  Delay1 : Delay  DelayLength=1  InitialCondition=0
  Delay2 : Delay  DelayLength=1  InitialCondition=0
  Delay4 : Delay  DelayLength=1  InitialCondition=0
  Digital Filter : Subsystem
  K1 : Gain  Gain=K1  OutDataTypeStr=fixdt(1,40,33)
  K2 : Gain  Gain=K2
  Sum2 : Sum  SaturateOnIntegerOverflow=on  InputSameDT=on
  v : Outport
  wires:
  e/1 -> Delay2/1
  Sum2/1 -> Data Type Conversion17/1
  Delay1/1 -> Sum2/1
  Delay4/1 -> Sum2/2
  Delay2/1 -> K1/1, K2/1
  Data Type Conversion17/1 -> v/1
  K2/1 -> Digital Filter/1(In1)
  Digital Filter/1(Out1) -> Delay4/1
  K1/1 -> Delay1/1

== system sdrzQPSKRxFPGA/QPSK Receiver/HDLRx/Coarse Frequency Compensation/luise_fixpt/Enabled Wire ==
  In1 : Inport
  Enable : EnablePort
  Data Type Conversion : DataTypeConversion  OutDataTypeStr=fixdt(1,sdrzQPSKrxFPGA.rad_WL,sdrzQPSKrxFPGA.rad_FL)
  Out1 : Outport  InitialOutput=0
  wires:
  Data Type Conversion/1 -> Out1/1
  In1/1 -> Data Type Conversion/1

== system sdrzQPSKRxFPGA/QPSK Receiver/HDLRx/Fine Frequency Compensation/Loop Filter/Digital Filter ==
  In1 : Inport
  Add1 : Sum  OutDataTypeStr=fixdt(1,32,29)
  Unit Delay1 : UnitDelay  SampleTime=-1
  Out1 : Outport
  wires:
  In1/1 -> Add1/2
  Add1/1 -> Unit Delay1/1, Out1/1
  Unit Delay1/1 -> Add1/1

== system sdrzQPSKRxFPGA/QPSK Receiver/HDLRx/Timing Recovery/Loop Filter/Digital Filter ==
  In1 : Inport
  Add2 : Sum  OutDataTypeStr=fixdt(1,40,33)
  Unit Delay1 : UnitDelay  SampleTime=-1
  Out1 : Outport
  wires:
  In1/1 -> Add2/2
  Add2/1 -> Unit Delay1/1, Out1/1
  Unit Delay1/1 -> Add2/1

== matlab function sdrzQPSKRxFPGA/QPSK Receiver/  ==
  data: RxGo output; framed_data output; bit1 input; bit2 input; datavld input
function [RxGo, framed_data] = dataframer(bit1, bit2, datavld)
%#codegen

persistent  gooddata_from_prev length_prev_good_data


if isempty(gooddata_from_prev)
    gooddata_from_prev = false(8000,1);
    length_prev_good_data = 0;
end

gooddata_current = false(8000,1); % worst case scenario
if any(datavld) % there is some valid data
    % get the valid data from this frame and append it with the previous
    % stored one, if any
    
    %gooddata_current = false(2*sum(datavld),1);
    gooddata_current(1:2:2*sum(datavld)-1) = bit1(logical(datavld));
    gooddata_current(2:2:2*sum(datavld))   = bit2(logical(datavld));
    % append with prev good data
    data_tmp = [gooddata_from_prev(1:length_prev_good_data);gooddata_current(1:2*sum(datavld))];
    if length(data_tmp) > 8000
        framed_data = data_tmp(1:8000);
        RxGo = 1;
        gooddata_length_athand = length(data_tmp);
        datalen_fornext = gooddata_length_athand -8000;
        gooddata_from_prev(1:datalen_fornext) = data_tmp(8001:8001+datalen_fornext-1);
        length_prev_good_data = datalen_fornext;
    elseif length(data_tmp) == 8000
        framed_data = data_tmp(1:8000);
        RxGo = 1;
        gooddata_from_prev =  false(8000,1);
        length_prev_good_data = 0;
    else % less than 8000
        gooddata_length_athand = length(data_tmp);
        datalen_fornext = gooddata_length_athand;      
        gooddata_from_prev(1:gooddata_length_athand) = data_tmp(1:gooddata_length_athand);
        length_prev_good_data = datalen_fornext;
        framed_data = false(8000,1); % garbage
        RxGo = 0;
    end
    
else % none of the data is valid
    RxGo = 0;
    framed_data = false(8000,1); %just send the data through
    gooddata_from_prev = false(8000,1);
    length_prev_good_data = 0;
end

== matlab function sdrzQPSKRxFPGA/QPSK Receiver/Descramble and Print/BitsToDecimal1 ==
  data: u input
function BitsToASCII(u)
% Convert bits to ASCII message.

persistent package_counter;
persistent error_counter;
if isempty(package_counter)
    package_counter = 0;
    error_counter   = 0;
end

coder.extrinsic('disp')
coder.extrinsic('num2str')

aa = de2bi(int8('Hello world 0'),7,'left-msb');
bits_ref = double(reshape(aa.',1,[]));
bits_ref = bits_ref(:);

error_counter   = error_counter   + sum(abs(bits_ref - u(1:91)));
package_counter = package_counter + 1;

% Convert binary-valued column vector to 7-bit decimal values.
w = [64 32 16 8 4 2 1]; % binary digit weighting
Nbits = numel(u);
Ny = Nbits/7;
y = zeros(1,Ny);
for i = 0:Ny-1
    y(i+1) = w*u(7*i+(1:7));
end

% Display ASCII message to command window
disp(char(y));

== matlab function sdrzQPSKRxFPGA/QPSK Receiver/HDLRx/Data Decoding/MATLAB Function3 ==
  data: dvalid output; Freeze_MF_Conj output; enable input; MF_Conj input
function [dvalid,Freeze_MF_Conj] = fcn(enable,MF_Conj)
%#codegen

persistent state;
persistent counter;
persistent MF_Out_Reg;

if isempty(state);
    state      = false;
    counter    = uint8(0);
    MF_Out_Reg = complex(fi(0,1,16,10),fi(0,1,16,10));
end

Freeze_MF_Conj = MF_Out_Reg;

if state==false
    dvalid=false;
else %state==true
    dvalid=true;
    counter = counter-1;         
end


% state transition
if state==false && enable==true
    state=true;
    counter=uint8(100);
    MF_Out_Reg=MF_Conj;
elseif state==true && counter==0
    if enable==true % packages come back-to-back
        state      = true;
        counter    = uint8(100);
        MF_Out_Reg = MF_Conj;
    else
        state = false;    
    end
end

== matlab function sdrzQPSKRxFPGA/QPSK Receiver/HDLRx/Fine Frequency Compensation/MATLAB Function1 ==
  data: In input; e output
function e  = PED(In)
% Input:
%   In - Input samples, oversampled by two
% Output:
%   e - Phase error
% PED implements 
% e = sign(real(In)).*imag(In) - sign(imag(In)).*real(In);

%#codegen

OP2 = real(In);
OP1 = imag(In);

Real = OP2;
Imag = OP1;

if (bitget(Real,16)==true) % real component is negative
    OP1 = fi(-Imag,1,16,14);
end
if (bitget(Imag,16)==true) % imaginary component is negative
    OP2 = fi(-Real,1,16,14);
end

e= fi(OP1-OP2,1,16,14);

== matlab function sdrzQPSKRxFPGA/QPSK Receiver/HDLRx/Timing Recovery/Interpolation Control ==
  data: Delta input; Underflow output; mu output
function [Underflow, mu] = Interpolation_ctrl(Delta)
% Implementation of modulo-1 counter for interpolation control listed in
% Figure 8.4.19 of "Digital Communications - A Discrete-Time Approach"
% by Michael Rice. See design details in Chapter 8.4.3 of the same book.
% 
% Input:
%   Delta - Loop filter output. If loop is in lock, delta would be small
%   qpsktxrx - Simulation parameter structure
% Output:
%   Underflow - Indicator of counter underflow. This is the strobe signal
%   for downstream processing
%   mu - Difference between actual sampling instant and the optimal instant,
%        between zero and one
%#codegen

% delay1 - Counter value delayed by 1 sample
% Regtemp - The estimated timing error normalized by half QPSK symbols

persistent delay1 Regtemp;  
if isempty(delay1)
    delay1  = fi(0,1,11,10);
    Regtemp = fi(0,1,11,10);
end

mask = fi(1-2^(-10),1,11,10);

counter = bitand(mask,delay1)-Delta-0.5; % decrementing counter
% if delay1 is a nonnegative number, 
% then mod(delay1,1) equals the fractional part of delay1

if counter < 0
    Underflow = true;
    Regtemp = bitshift(bitand(mask,delay1),1);     
else
    Underflow = false;
end

mu = Regtemp;

% Update delay buffer
if counter<0
    delay1 = fi(counter+1,1,11,10); %make sure delay1 stays nonnegative
else
    delay1 = fi(counter,1,11,10);
end

== matlab function sdrzQPSKRxFPGA/QPSK Receiver/HDLRx/Timing Recovery/Timing Error Detector ==
  data: In input; strobe input; e output
function e = TED(In, strobe)
% Zero-Crossing Timing Error Detector. See "Zero-Crossing Timing Error
% Detector" section in Chapter 8.4.1 of "Digital Communications - A
% Discrete-Time Approach" by Michael Rice. For bit stuffing/stripping
% details, see page 490-494 of the same book.
%
% Input: 
%   In - Input samples, interpolation result
%   strobe - Signal to enable timing error calculation
% Output:
%   e - Timing error
%#codegen

persistent delay1_R delay1_I delay2_R delay2_I delayStrobe; 
% Input delayed by one and 2 samples, and
% Enable signal delayed by one sample
if isempty(delay1_R)    
    delay1_R=fi(0,1,16,10);
    delay1_I=fi(0,1,16,10);
    delay2_R=fi(0,1,16,10);
    delay2_I=fi(0,1,16,10);    
    delayStrobe = false;
end

In_Real = real(In);
In_Imag = imag(In);

if strobe==true && delayStrobe~=strobe
    if ( bitget(delay2_R,16)==bitget(In_Real,16) )         
        OP1=fi(0,1,16,10);
    elseif bitget(delay2_R,16)==true         
        OP1=fi(-1*bitshift(delay1_R,1),1,16,10);
    else        
        OP1=fi(bitshift(delay1_R,1),1,16,10);
    end
    
    if ( bitget(delay2_I,16)==bitget(In_Imag,16) )        
        OP2=fi(0,1,16,10);
    elseif bitget(delay2_I,16)==true        
        OP2=fi(-1*bitshift(delay1_I,1),1,16,10);
    else        
        OP2=fi(bitshift(delay1_I,1),1,16,10);
    end
else
    OP1=fi(0,1,16,10);
    OP2=fi(0,1,16,10);
end

e = fi(OP1+OP2,1,16,10);


if delayStrobe~=strobe
    % Shift contents in delay register
    delay2_R = delay1_R;
    delay1_R = In_Real;
    delay2_I = delay1_I;
    delay1_I = In_Imag;
elseif strobe==true
    % Two consecutive high strobes
    delay2_R = fi(0,1,16,10); % Stuff missing sample
    delay1_R = In_Real; 
    delay2_I = fi(0,1,16,10); % Stuff missing sample
    delay1_I = In_Imag; 
end

% If both current and previous enable signals are 0, skip current sample
% and keep the delayed signals unchanged. (Bit stripping)
delayStrobe = strobe;
